simulink model "modelo_NL_DH_CL"  (R2025b)
settings: Solver=ode4  StartTime=0.0  StopTime=60  FixedStep=SampleTime  RelTol=1e-3
undefined symbols (not defined in the file): act, C_alt, C_phi, C_theta, C_vel, eng, h_ref, h_step_final, h_step_init, h_step_t, h_step_t2, h_step_t3, he, K_heading, Kp, Kq, Kr, psi_ref_final, psi_ref_init, psi_ref_t, psi_ref_t2, psi_ref_t3, tau_ref, theta_ref_clamp, TrimInput, Ue, Ve, VT_ref, VT_step_delta, VT_step_t, Xe
libraries: slpidlib x4
settings Model: Creator=anade  LastModifiedBy=kaue
settings SolverCC: ZeroCrossAlgorithm=Adaptive
settings DebuggingCC: AlgebraicLoopMsg=none  IgnoredZcDiagnostic=none

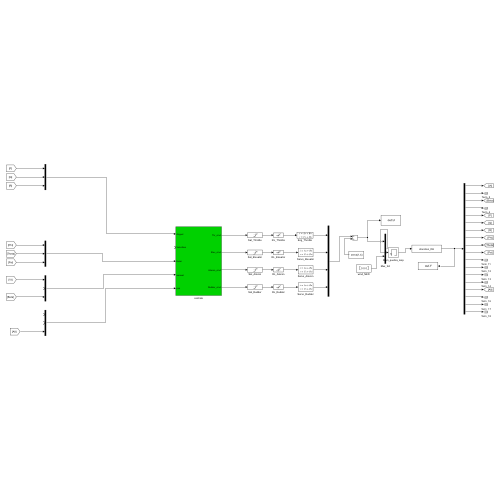
[thumbnail: Simulink's stored preview of the top-level diagram]
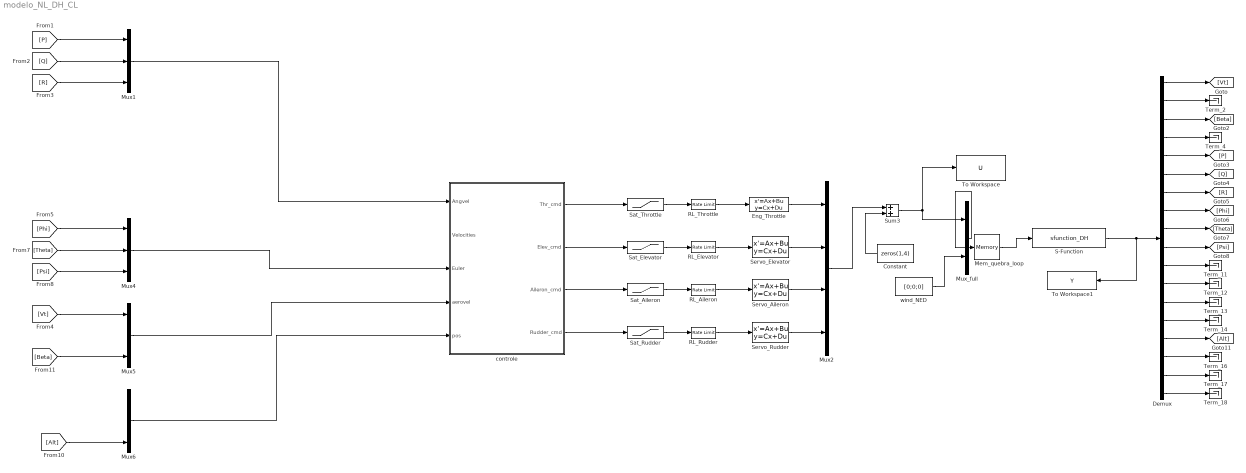
== system modelo_NL_DH_CL ==
  Constant : Constant  Value=zeros(1,4)
  Demux : Demux  Outputs=18
  Eng_Throttle : StateSpace  A=-1/eng.tau  B=1/eng.tau  D=0  InitialCondition=TrimInput(1)
  Mem_quebra_loop : Memory  Description=Quebra o loop algebrico da malha de controle atraves da S-function nivel-1 (que declara feedthrough direto em todas as entradas). Atraso de 1 passo (0.01 s) = comportamento do firmware real a 100 Hz, que atua com a medicao do ciclo anterior. IC = Ue (trim 7 entradas: 4 superficies + vento NED zero), sem transiente em t=0. Ganho medido: sim de 60 s caiu de ~100 s para ~9 s, diferenca de trajetoria <=0.18 deg / 1.1 cm na manobra agressiva (2026-06-09).  InitialCondition=Ue
  Mux{1,4..6} (4 alike) : Mux  Inputs=3
  Mux2 : Mux
  Mux_full : Mux  Inputs=2
  RL_Aileron : RateLimiter  RisingSlewLimit=act.rate  FallingSlewLimit=-act.rate  InitialCondition=TrimInput(3)
  RL_Elevator : RateLimiter  RisingSlewLimit=act.rate  FallingSlewLimit=-act.rate  InitialCondition=TrimInput(2)
  RL_Rudder : RateLimiter  RisingSlewLimit=act.rate  FallingSlewLimit=-act.rate  InitialCondition=TrimInput(4)
  RL_Throttle : RateLimiter  RisingSlewLimit=eng.rate  FallingSlewLimit=-eng.rate  InitialCondition=TrimInput(1)
  S-Function : S-Function  FunctionName=sfunction_DH  Parameters=Xe  SFunctionDeploymentMode=off  EnableBusSupport=off
  Sat_Aileron : Saturate  UpperLimit=0.4363  LowerLimit=-0.4363
  Sat_Elevator : Saturate  UpperLimit=0.4363  LowerLimit=-0.4363
  Sat_Rudder : Saturate  UpperLimit=0.4363  LowerLimit=-0.4363
  Sat_Throttle : Saturate  UpperLimit=1  LowerLimit=0
  Servo_Aileron : StateSpace  A=-act.bw  B=act.bw  D=0  InitialCondition=TrimInput(3)
  Servo_Elevator : StateSpace  A=-act.bw  B=act.bw  D=0  InitialCondition=TrimInput(2)
  Servo_Rudder : StateSpace  A=-act.bw  B=act.bw  D=0  InitialCondition=TrimInput(4)
  Sum3 : Sum
  Term_{2,4,11..14,16..18} (9 alike) : Terminator
  To Workspace : ToWorkspace  VariableName=U  SaveFormat=Structure With Time  SampleTime=-1
  To Workspace1 : ToWorkspace  VariableName=Y  SaveFormat=Structure With Time  SampleTime=-1
  controle : Subsystem
  wind_NED : Constant  Value=[0;0;0]
  wires:
  [Theta] -> Mux4/2
  Mux1/1 -> controle/1(Angvel)
  [Alt] -> Mux6/3
  [P] -> Mux1/1
  Mux4/1 -> controle/3(Euler)
  [R] -> Mux1/3
  [Phi] -> Mux4/1
  Mux6/1 -> controle/5(pos)
  [Q] -> Mux1/2
  Mux5/1 -> controle/4(aerovel)
  [Psi] -> Mux4/3
  [Beta] -> Mux5/3
  [Vt] -> Mux5/1
  controle/1(Thr_cmd) -> Sat_Throttle/1
  controle/2(Elev_cmd) -> Sat_Elevator/1
  controle/3(Aileron_cmd) -> Sat_Aileron/1
  controle/4(Rudder_cmd) -> Sat_Rudder/1
  Mux2/1 -> Sum3/1
  Constant/1 -> Sum3/2
  Sum3/1 -> Mux_full/1, To Workspace/1
  wind_NED/1 -> Mux_full/2
  S-Function/1 -> Demux/1, To Workspace1/1
  Demux/1 -> [Vt]
  Demux/2 -> Term_2/1
  Demux/3 -> [Beta]
  Demux/4 -> Term_4/1
  Demux/5 -> [P]
  Demux/6 -> [Q]
  Demux/7 -> [R]
  Demux/8 -> [Phi]
  Demux/9 -> [Theta]
  Demux/10 -> [Psi]
  Demux/11 -> Term_11/1
  Demux/12 -> Term_12/1
  Demux/13 -> Term_13/1
  Demux/14 -> Term_14/1
  Demux/15 -> [Alt]
  Demux/16 -> Term_16/1
  Demux/17 -> Term_17/1
  Demux/18 -> Term_18/1
  Mux_full/1 -> Mem_quebra_loop/1
  Mem_quebra_loop/1 -> S-Function/1
  Sat_Elevator/1 -> RL_Elevator/1
  Sat_Aileron/1 -> RL_Aileron/1
  Sat_Rudder/1 -> RL_Rudder/1
  RL_Elevator/1 -> Servo_Elevator/1
  Servo_Elevator/1 -> Mux2/2
  RL_Aileron/1 -> Servo_Aileron/1
  Servo_Aileron/1 -> Mux2/3
  RL_Rudder/1 -> Servo_Rudder/1
  Servo_Rudder/1 -> Mux2/4
  Sat_Throttle/1 -> RL_Throttle/1
  RL_Throttle/1 -> Eng_Throttle/1
  Eng_Throttle/1 -> Mux2/1

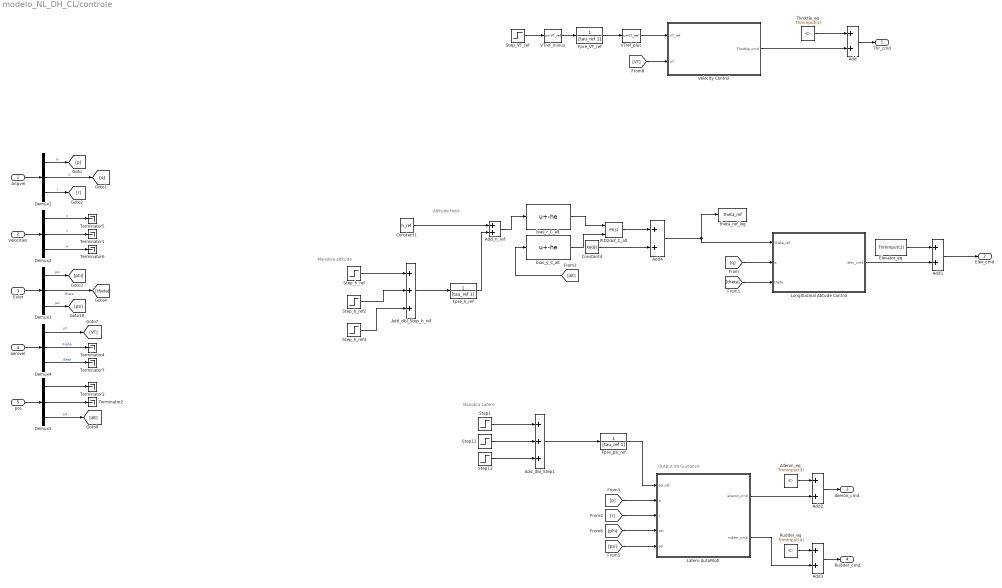
== system modelo_NL_DH_CL/controle ==
  note: Manobra
      | Latero
  note: Manobra
      | altitude
  note: Altitude Hold
  note: Output do Guidance
  Angvel : Inport
  Velocities : Inport  Port=2
  Euler : Inport  Port=3
  aerovel : Inport  Port=4
  pos : Inport  Port=5
  Add{,1..4} (5 alike) : Sum
  Add_dbl_Step1 : Sum  Inputs=+++
  Add_dbl_Step_h_ref : Sum  Inputs=+++
  Add_h_ref : Sum
  Aileron_eq : Constant  Value=TrimInput(3)
  Constant1 : Constant  Value=h_ref
  Constant4 : Constant  Value=Xe(8)
  Demux{1..5} (5 alike) : Demux  Outputs=3
  Elevator_eq : Constant  Value=TrimInput(2)
  Fpre_VT_ref : TransferFcn  Denominator=[tau_ref 1]
  Fpre_h_ref : TransferFcn  Denominator=[tau_ref 1]
  Fpre_psi_ref : TransferFcn  Denominator=[tau_ref 1]
  Latero AutoPilotl : Subsystem
  Longitudinal Atitude Control : Subsystem
  PID2dof_C_alt : slpidlib/PID Controller (2DOF)  Controller=PI  Form=Parallel  TimeDomain=Continuous-time  UseExternalTs=off  SampleTime=-1  IntegratorMethod=Forward Euler  FilterMethod=Forward Euler  ControllerParametersSource=internal  P=C_alt.Kp  I=C_alt.Ki  UseKiTs=off  D=0  UseExternalDerivativeSource=off  N=100  UseFilter=on  b=0  c=1  TunerSelectOption=Transfer Function Based (PID Tuner App)  InitialConditionSource=internal  InitialConditionForIntegrator=0  InitialConditionForFilter=0  DifferentiatorICPrevScaledInput=0  ExternalReset=none  TrackingMode=off  Kt=1  LimitOutput=on  SatLimitsSource=internal  UpperSaturationLimit=theta_ref_clamp(2)  LowerSaturationLimit=theta_ref_clamp(1)  LinearizeAsGain=on  AntiWindupMode=clamping  Kb=1  LimitIntegrator=off  UpperIntegratorSaturationLimit=inf  LowerIntegratorSaturationLimit=-inf  POutMin=[]  POutMax=[]  IOutMin=[]  IOutMax=[]  DOutMin=[]  DOutMax=[]  NOutMin=[]  NOutMax=[]  bOutMin=[]  bOutMax=[]  cOutMin=[]  cOutMax=[]  SumOutMin=[]  SumOutMax=[]  SaturationOutMin=[]  SaturationOutMax=[]  PParamMin=[]  PParamMax=[]  IParamMin=[]  IParamMax=[]  DParamMin=[]  DParamMax=[]  NParamMin=[]  NParamMax=[]  bParamMin=[]  bParamMax=[]  cParamMin=[]  cParamMax=[]  KbParamMin=[]  KbParamMax=[]  KtParamMin=[]  KtParamMax=[]  KbOutMin=[]  KbOutMax=[]  KtOutMin=[]  KtOutMax=[]  IntegratorOutMin=[]  IntegratorOutMax=[]  FilterOutMin=[]  FilterOutMax=[]  SumI1OutMin=[]  SumI1OutMax=[]  SumI2OutMin=[]  SumI2OutMax=[]  SumI3OutMin=[]  SumI3OutMax=[]  SumI4OutMin=[]  SumI4OutMax=[]  SumDOutMin=[]  SumDOutMax=[]  Sum1OutMin=[]  Sum1OutMax=[]  Sum2OutMin=[]  Sum2OutMax=[]  Sum3OutMin=[]  Sum3OutMax=[]  DifferentiatorOutMin=[]  DifferentiatorOutMax=[]  FilterDiffOutCoefMin=[]  FilterDiffOutCoefMax=[]  ReciprocalOutMin=[]  ReciprocalOutMax=[]  SumDenOutMin=[]  SumDenOutMax=[]  SumNumOutMin=[]  SumNumOutMax=[]  DivideOutMin=[]  DivideOutMax=[]  UdiffTsProdOutMin=[]  UdiffTsProdOutMax=[]  NTsProdOutMin=[]  NTsProdOutMax=[]  UintegralTsProdOutMin=[]  UintegralTsProdOutMax=[]  UngainTsProdOutMin=[]  UngainTsProdOutMax=[]  ClampingZeroOutDataTypeStr=Inherit: Inherit via back propagation  ClampingZeroOutMin=[]  ClampingZeroOutMax=[]  FilterDenConstantOutDataTypeStr=Inherit: Inherit via back propagation  FilterDenConstantOutMin=[]  FilterDenConstantOutMax=[]  PCopyOutDataTypeStr=Inherit: Inherit via back propagation  PCopyOutMin=[]  PCopyOutMax=[]  NCopyOutDataTypeStr=Inherit: Inherit via back propagation  NCopyOutMin=[]  NCopyOutMax=[]  IntegratorContinuousStateAttributes=''  IntegratorStateMustResolveToSignalObject=off  IntegratorRTWStateStorageClass=Auto  FilterContinuousStateAttributes=''  FilterStateMustResolveToSignalObject=off  FilterRTWStateStorageClass=Auto  ParallelPVariant=InternalParameters  IdealPVariant=Disabled  IVariant=InternalParameters  DVariant=Disabled  bVariant=InternalParameters  cVariant=Disabled  IntegratorVariant=Continuous  SatVariant=Enabled  AWVariant=ContClampingParallel  PCopyVariant=Disabled  TRVariant=Disabled  FdbkBlocksVariant=Forward  IdealPFdbkVariant=Disabled  SatFdbkVariant=Disabled  DerivativeFilterVariant=Disabled  NVariant=Disabled  NCopyVariant=Disabled_SignalSpec  FilterICVariant=Disabled  IntegratorICVariant=InternalICs  ExternalResetVariant=Disabled  TRSumVariant=Passthrough  SumFdbkVariant=Disabled  SumVariant=Sum_PI  TsampFilterVariant=InternalTs  TsampNgainVariant=Passthrough  TsampIntegralVariant=Disabled_SignalSpec  ExternalSaturationOutDataTypeStr=Inherit: Same as second input  DerivativeSourceVariant=Disabled  PreIntVariant=InternalPreInt
  Rudder_eq : Constant  Value=TrimInput(4)
  Step1 : Step  Time=psi_ref_t  Before=psi_ref_init  After=psi_ref_final  SampleTime=0
  Step12 : Step  Time=psi_ref_t2  After=-2*psi_ref_final  SampleTime=0
  Step13 : Step  Time=psi_ref_t3  After=psi_ref_final  SampleTime=0
  Step_VT_ref : Step  Time=VT_step_t  Before=VT_ref  After=VT_ref+VT_step_delta  SampleTime=0
  Step_h_ref : Step  Time=h_step_t  Before=h_step_init  After=h_step_final  SampleTime=0
  Step_h_ref2 : Step  Time=h_step_t2  After=-2*h_step_final  SampleTime=0
  Step_h_ref3 : Step  Time=h_step_t3  After=h_step_final  SampleTime=0
  Terminator{1..7} (7 alike) : Terminator
  Throttle_eq : Constant  Value=TrimInput(1)
  VTref_minus : Bias  Bias=-VT_ref
  VTref_plus : Bias  Bias=VT_ref
  Velocity Control : Subsystem
  bias_r_C_alt : Bias  Bias=-he  SaturateOnIntegerOverflow=off
  bias_y_C_alt : Bias  Bias=-he  SaturateOnIntegerOverflow=off
  theta_ref_log : ToWorkspace  VariableName=theta_ref  SaveFormat=Structure With Time  SampleTime=-1
  Thr_cmd : Outport
  Elev_cmd : Outport  Port=2
  Aileron_cmd : Outport  Port=3
  Rudder_cmd : Outport  Port=4
  wires:
  Angvel/1 -> Demux1/1
  Velocities/1 -> Demux2/1
  Demux1/1 -> [p]  "p"
  Demux1/2 -> [q]  "q"
  Demux1/3 -> [r]  "r"
  Euler/1 -> Demux3/1
  Demux3/3 -> [psi]  "psi"
  Demux3/1 -> [phi]  "phi"
  Demux3/2 -> [theta]  "theta"
  Demux2/3 -> Terminator6/1  "w"
  Demux2/1 -> Terminator5/1  "u"
  Demux2/2 -> Terminator1/1  "v"
  [theta] -> Longitudinal Atitude Control/3(theta)
  aerovel/1 -> Demux4/1
  Demux4/1 -> [VT]  "VT"
  Demux4/2 -> Terminator4/1  "Alpha"
  Demux4/3 -> Terminator7/1  "Beta"
  [q] -> Longitudinal Atitude Control/2(q)
  [VT] -> Velocity Control/2(VT)
  pos/1 -> Demux5/1
  Demux5/3 -> [alt]  "alt"
  Demux5/2 -> Terminator2/1
  Demux5/1 -> Terminator3/1
  [p] -> Latero AutoPilotl/2(p)
  [r] -> Latero AutoPilotl/3(r)
  [psi] -> Latero AutoPilotl/5(psi)
  [phi] -> Latero AutoPilotl/4(phi)
  Constant4/1 -> Add4/2
  Add1/1 -> Elev_cmd/1
  Longitudinal Atitude Control/1(elev_cmd) -> Add1/2
  Add/1 -> Thr_cmd/1
  Velocity Control/1(Throttle_cmd) -> Add/2
  Latero AutoPilotl/1(aileron_cmd) -> Add2/2
  Elevator_eq/1 -> Add1/1
  Rudder_eq/1 -> Add3/1
  Aileron_eq/1 -> Add2/1
  Latero AutoPilotl/2(rudder_cmd) -> Add3/2
  Add2/1 -> Aileron_cmd/1
  Add3/1 -> Rudder_cmd/1
  Throttle_eq/1 -> Add/1
  Step_VT_ref/1 -> VTref_minus/1
  Add4/1 -> theta_ref_log/1, Longitudinal Atitude Control/1(Theta_ref)
  Constant1/1 -> Add_h_ref/1
  Step_h_ref/1 -> Add_dbl_Step_h_ref/1
  Step_h_ref2/1 -> Add_dbl_Step_h_ref/2
  Step_h_ref3/1 -> Add_dbl_Step_h_ref/3
  Step1/1 -> Add_dbl_Step1/1
  Step12/1 -> Add_dbl_Step1/2
  Step13/1 -> Add_dbl_Step1/3
  Add_dbl_Step_h_ref/1 -> Fpre_h_ref/1
  Fpre_h_ref/1 -> Add_h_ref/2
  Add_dbl_Step1/1 -> Fpre_psi_ref/1
  Fpre_psi_ref/1 -> Latero AutoPilotl/1(psi_ref)
  VTref_minus/1 -> Fpre_VT_ref/1
  Fpre_VT_ref/1 -> VTref_plus/1
  VTref_plus/1 -> Velocity Control/1(VT_ref)
  Add_h_ref/1 -> bias_r_C_alt/1
  [alt] -> bias_y_C_alt/1
  bias_r_C_alt/1 -> PID2dof_C_alt/1
  bias_y_C_alt/1 -> PID2dof_C_alt/2
  PID2dof_C_alt/1 -> Add4/1

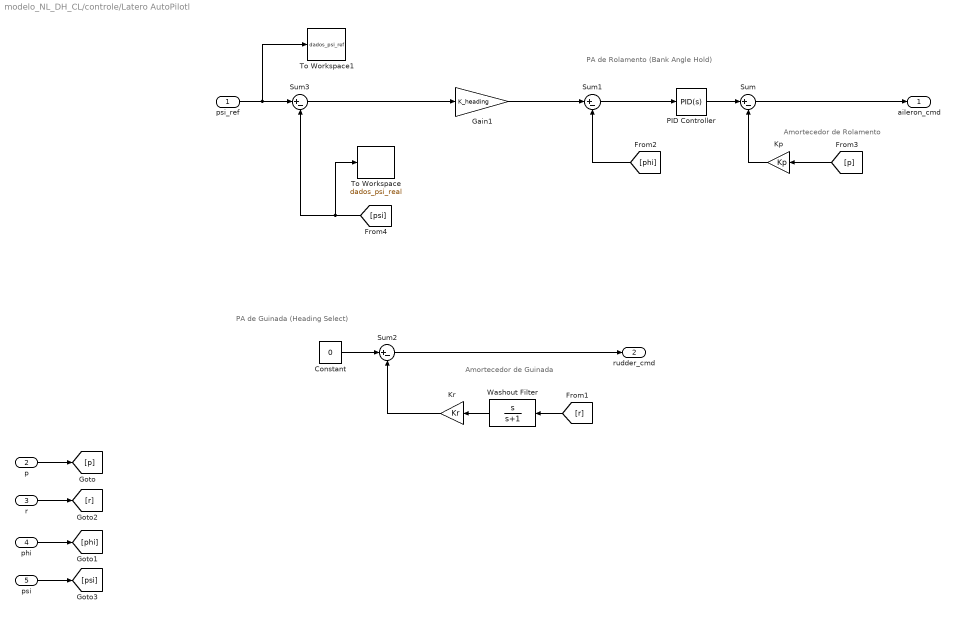
== system modelo_NL_DH_CL/controle/Latero AutoPilotl ==
  note: PA de Rolamento (Bank Angle Hold)
  note: Amortecedor de Rolamento
  note: Amortecedor de Guinada
  note: PA de Guinada (Heading Select)
  psi_ref : Inport
  p : Inport  Port=2
  r : Inport  Port=3
  phi : Inport  Port=4
  psi : Inport  Port=5
  Constant : Constant  Value=0
  Gain1 : Gain  Gain=K_heading
  Kp : Gain  Gain=Kp
  Kr : Gain  Gain=Kr
  PID Controller : slpidlib/PID Controller  Controller=PID  Form=Parallel  TimeDomain=Continuous-time  UseExternalTs=off  SampleTime=-1  IntegratorMethod=Forward Euler  FilterMethod=Forward Euler  ControllerParametersSource=internal  P=C_phi.Kp  I=C_phi.Ki  UseKiTs=off  D=C_phi.Kd  UseExternalDerivativeSource=off  N=C_phi.N  UseFilter=on  TunerSelectOption=Transfer Function Based (PID Tuner App)  InitialConditionSource=internal  InitialConditionForIntegrator=0  InitialConditionForFilter=0  DifferentiatorICPrevScaledInput=0  ExternalReset=none  TrackingMode=off  Kt=1  LimitOutput=on  SatLimitsSource=internal  UpperSaturationLimit=0.4363  LowerSaturationLimit=-0.4363  LinearizeAsGain=on  AntiWindupMode=clamping  Kb=1  LimitIntegrator=off  UpperIntegratorSaturationLimit=inf  LowerIntegratorSaturationLimit=-inf  POutMin=[]  POutMax=[]  IOutMin=[]  IOutMax=[]  DOutMin=[]  DOutMax=[]  NOutMin=[]  NOutMax=[]  SumOutMin=[]  SumOutMax=[]  SaturationOutMin=[]  SaturationOutMax=[]  PParamMin=[]  PParamMax=[]  IParamMin=[]  IParamMax=[]  DParamMin=[]  DParamMax=[]  NParamMin=[]  NParamMax=[]  KbParamMin=[]  KbParamMax=[]  KtParamMin=[]  KtParamMax=[]  KbOutMin=[]  KbOutMax=[]  KtOutMin=[]  KtOutMax=[]  IntegratorOutMin=[]  IntegratorOutMax=[]  FilterOutMin=[]  FilterOutMax=[]  SumI1OutMin=[]  SumI1OutMax=[]  SumI2OutMin=[]  SumI2OutMax=[]  SumI3OutMin=[]  SumI3OutMax=[]  SumI4OutMin=[]  SumI4OutMax=[]  SumDOutMin=[]  SumDOutMax=[]  DifferentiatorOutMin=[]  DifferentiatorOutMax=[]  FilterDiffOutCoefMin=[]  FilterDiffOutCoefMax=[]  ReciprocalOutMin=[]  ReciprocalOutMax=[]  SumDenOutMin=[]  SumDenOutMax=[]  SumNumOutMin=[]  SumNumOutMax=[]  DivideOutMin=[]  DivideOutMax=[]  UdiffTsProdOutMin=[]  UdiffTsProdOutMax=[]  NTsProdOutMin=[]  NTsProdOutMax=[]  UintegralTsProdOutMin=[]  UintegralTsProdOutMax=[]  UngainTsProdOutMin=[]  UngainTsProdOutMax=[]  ClampingZeroOutDataTypeStr=Inherit: Inherit via back propagation  ClampingZeroOutMin=[]  ClampingZeroOutMax=[]  FilterDenConstantOutDataTypeStr=Inherit: Inherit via back propagation  FilterDenConstantOutMin=[]  FilterDenConstantOutMax=[]  PCopyOutDataTypeStr=Inherit: Inherit via back propagation  PCopyOutMin=[]  PCopyOutMax=[]  NCopyOutDataTypeStr=Inherit: Inherit via back propagation  NCopyOutMin=[]  NCopyOutMax=[]  IntegratorContinuousStateAttributes=''  IntegratorStateMustResolveToSignalObject=off  IntegratorRTWStateStorageClass=Auto  FilterContinuousStateAttributes=''  FilterStateMustResolveToSignalObject=off  FilterRTWStateStorageClass=Auto  ParallelPVariant=InternalParameters  IdealPVariant=Disabled  IVariant=InternalParameters  DVariant=InternalParameters  IntegratorVariant=Continuous  SatVariant=Enabled  AWVariant=ContClampingParallel  PCopyVariant=Disabled  TRVariant=Disabled  FdbkBlocksVariant=Forward  IdealPFdbkVariant=Disabled  SatFdbkVariant=Disabled  DerivativeFilterVariant=ContFilter  NVariant=InternalParameters  NCopyVariant=Disabled  FilterICVariant=InternalICsFilter  IntegratorICVariant=InternalICs  ExternalResetVariant=Disabled  TRSumVariant=Passthrough  SumFdbkVariant=Disabled  SumVariant=Sum_PID  TsampFilterVariant=InternalTs  TsampNgainVariant=Passthrough  TsampIntegralVariant=Disabled_SignalSpec  ExternalSaturationOutDataTypeStr=Inherit: Same as second input  DerivativeSourceVariant=ErrorSignal  PreIntVariant=InternalPreInt
  Sum{,1..3} (4 alike) : Sum  Inputs=|+-
  To Workspace : ToWorkspace  VariableName=dados_psi_real  SaveFormat=Timeseries  SampleTime=-1
      settings: Save2DSignal=2-D array (concatenate along first dimension)
  To Workspace1 : ToWorkspace  VariableName=dados_psi_ref  SaveFormat=Timeseries  SampleTime=-1
      settings: Save2DSignal=2-D array (concatenate along first dimension)
  Washout Filter : TransferFcn  Numerator=[1 0]  Denominator=[1 1]
  aileron_cmd : Outport
  rudder_cmd : Outport  Port=2
  wires:
  [p] -> Kp/1
  [phi] -> Sum1/2
  Kp/1 -> Sum/2
  PID Controller/1 -> Sum/1
  p/1 -> [p]
  [r] -> Washout Filter/1
  Kr/1 -> Sum2/2
  r/1 -> [r]
  Washout Filter/1 -> Kr/1
  phi/1 -> [phi]
  psi/1 -> [psi]
  Sum3/1 -> Gain1/1
  [psi] -> Sum3/2, To Workspace/1
  psi_ref/1 -> Sum3/1, To Workspace1/1
  Sum2/1 -> rudder_cmd/1
  Constant/1 -> Sum2/1
  Gain1/1 -> Sum1/1
  Sum/1 -> aileron_cmd/1
  Sum1/1 -> PID Controller/1

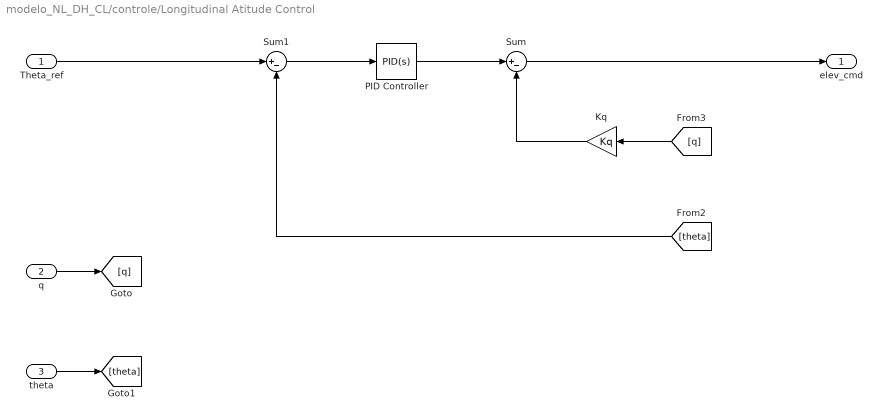
== system modelo_NL_DH_CL/controle/Longitudinal Atitude Control ==
  Theta_ref : Inport
  q : Inport  Port=2
  theta : Inport  Port=3
  Kq : Gain  Gain=Kq
  PID Controller : slpidlib/PID Controller  Controller=PID  Form=Parallel  TimeDomain=Continuous-time  UseExternalTs=off  SampleTime=-1  IntegratorMethod=Forward Euler  FilterMethod=Forward Euler  ControllerParametersSource=internal  P=C_theta.Kp  I=C_theta.Ki  UseKiTs=off  D=C_theta.Kd  UseExternalDerivativeSource=off  N=C_theta.N  UseFilter=on  TunerSelectOption=Transfer Function Based (PID Tuner App)  InitialConditionSource=internal  InitialConditionForIntegrator=0  InitialConditionForFilter=0  DifferentiatorICPrevScaledInput=0  ExternalReset=none  TrackingMode=off  Kt=1  LimitOutput=on  SatLimitsSource=internal  UpperSaturationLimit=0.4363  LowerSaturationLimit=-0.4363  LinearizeAsGain=on  AntiWindupMode=clamping  Kb=1  LimitIntegrator=off  UpperIntegratorSaturationLimit=inf  LowerIntegratorSaturationLimit=-inf  POutMin=[]  POutMax=[]  IOutMin=[]  IOutMax=[]  DOutMin=[]  DOutMax=[]  NOutMin=[]  NOutMax=[]  SumOutMin=[]  SumOutMax=[]  SaturationOutMin=[]  SaturationOutMax=[]  PParamMin=[]  PParamMax=[]  IParamMin=[]  IParamMax=[]  DParamMin=[]  DParamMax=[]  NParamMin=[]  NParamMax=[]  KbParamMin=[]  KbParamMax=[]  KtParamMin=[]  KtParamMax=[]  KbOutMin=[]  KbOutMax=[]  KtOutMin=[]  KtOutMax=[]  IntegratorOutMin=[]  IntegratorOutMax=[]  FilterOutMin=[]  FilterOutMax=[]  SumI1OutMin=[]  SumI1OutMax=[]  SumI2OutMin=[]  SumI2OutMax=[]  SumI3OutMin=[]  SumI3OutMax=[]  SumI4OutMin=[]  SumI4OutMax=[]  SumDOutMin=[]  SumDOutMax=[]  DifferentiatorOutMin=[]  DifferentiatorOutMax=[]  FilterDiffOutCoefMin=[]  FilterDiffOutCoefMax=[]  ReciprocalOutMin=[]  ReciprocalOutMax=[]  SumDenOutMin=[]  SumDenOutMax=[]  SumNumOutMin=[]  SumNumOutMax=[]  DivideOutMin=[]  DivideOutMax=[]  UdiffTsProdOutMin=[]  UdiffTsProdOutMax=[]  NTsProdOutMin=[]  NTsProdOutMax=[]  UintegralTsProdOutMin=[]  UintegralTsProdOutMax=[]  UngainTsProdOutMin=[]  UngainTsProdOutMax=[]  ClampingZeroOutDataTypeStr=Inherit: Inherit via back propagation  ClampingZeroOutMin=[]  ClampingZeroOutMax=[]  FilterDenConstantOutDataTypeStr=Inherit: Inherit via back propagation  FilterDenConstantOutMin=[]  FilterDenConstantOutMax=[]  PCopyOutDataTypeStr=Inherit: Inherit via back propagation  PCopyOutMin=[]  PCopyOutMax=[]  NCopyOutDataTypeStr=Inherit: Inherit via back propagation  NCopyOutMin=[]  NCopyOutMax=[]  IntegratorContinuousStateAttributes=''  IntegratorStateMustResolveToSignalObject=off  IntegratorRTWStateStorageClass=Auto  FilterContinuousStateAttributes=''  FilterStateMustResolveToSignalObject=off  FilterRTWStateStorageClass=Auto  ParallelPVariant=InternalParameters  IdealPVariant=Disabled  IVariant=InternalParameters  DVariant=InternalParameters  IntegratorVariant=Continuous  SatVariant=Enabled  AWVariant=ContClampingParallel  PCopyVariant=Disabled  TRVariant=Disabled  FdbkBlocksVariant=Forward  IdealPFdbkVariant=Disabled  SatFdbkVariant=Disabled  DerivativeFilterVariant=ContFilter  NVariant=InternalParameters  NCopyVariant=Disabled  FilterICVariant=InternalICsFilter  IntegratorICVariant=InternalICs  ExternalResetVariant=Disabled  TRSumVariant=Passthrough  SumFdbkVariant=Disabled  SumVariant=Sum_PID  TsampFilterVariant=InternalTs  TsampNgainVariant=Passthrough  TsampIntegralVariant=Disabled_SignalSpec  ExternalSaturationOutDataTypeStr=Inherit: Same as second input  DerivativeSourceVariant=ErrorSignal  PreIntVariant=InternalPreInt
  Sum : Sum  Inputs=|+-
  Sum1 : Sum  Inputs=|+-
  elev_cmd : Outport
  wires:
  Sum1/1 -> PID Controller/1
  Sum/1 -> elev_cmd/1
  [q] -> Kq/1
  [theta] -> Sum1/2
  Kq/1 -> Sum/2
  PID Controller/1 -> Sum/1
  theta/1 -> [theta]
  q/1 -> [q]
  Theta_ref/1 -> Sum1/1

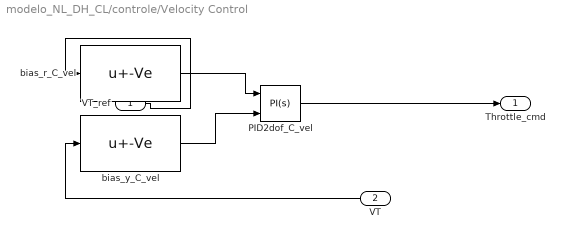
== system modelo_NL_DH_CL/controle/Velocity Control ==
  VT_ref : Inport
  VT : Inport  Port=2
  PID2dof_C_vel : slpidlib/PID Controller (2DOF)  Controller=PI  Form=Parallel  TimeDomain=Continuous-time  UseExternalTs=off  SampleTime=-1  IntegratorMethod=Forward Euler  FilterMethod=Forward Euler  ControllerParametersSource=internal  P=C_vel.Kp  I=C_vel.Ki  UseKiTs=off  D=0  UseExternalDerivativeSource=off  N=100  UseFilter=on  b=0  c=1  TunerSelectOption=Transfer Function Based (PID Tuner App)  InitialConditionSource=internal  InitialConditionForIntegrator=0  InitialConditionForFilter=0  DifferentiatorICPrevScaledInput=0  ExternalReset=none  TrackingMode=off  Kt=1  LimitOutput=on  SatLimitsSource=internal  UpperSaturationLimit=0.51  LowerSaturationLimit=-0.49  LinearizeAsGain=on  AntiWindupMode=clamping  Kb=1  LimitIntegrator=off  UpperIntegratorSaturationLimit=inf  LowerIntegratorSaturationLimit=-inf  POutMin=[]  POutMax=[]  IOutMin=[]  IOutMax=[]  DOutMin=[]  DOutMax=[]  NOutMin=[]  NOutMax=[]  bOutMin=[]  bOutMax=[]  cOutMin=[]  cOutMax=[]  SumOutMin=[]  SumOutMax=[]  SaturationOutMin=[]  SaturationOutMax=[]  PParamMin=[]  PParamMax=[]  IParamMin=[]  IParamMax=[]  DParamMin=[]  DParamMax=[]  NParamMin=[]  NParamMax=[]  bParamMin=[]  bParamMax=[]  cParamMin=[]  cParamMax=[]  KbParamMin=[]  KbParamMax=[]  KtParamMin=[]  KtParamMax=[]  KbOutMin=[]  KbOutMax=[]  KtOutMin=[]  KtOutMax=[]  IntegratorOutMin=[]  IntegratorOutMax=[]  FilterOutMin=[]  FilterOutMax=[]  SumI1OutMin=[]  SumI1OutMax=[]  SumI2OutMin=[]  SumI2OutMax=[]  SumI3OutMin=[]  SumI3OutMax=[]  SumI4OutMin=[]  SumI4OutMax=[]  SumDOutMin=[]  SumDOutMax=[]  Sum1OutMin=[]  Sum1OutMax=[]  Sum2OutMin=[]  Sum2OutMax=[]  Sum3OutMin=[]  Sum3OutMax=[]  DifferentiatorOutMin=[]  DifferentiatorOutMax=[]  FilterDiffOutCoefMin=[]  FilterDiffOutCoefMax=[]  ReciprocalOutMin=[]  ReciprocalOutMax=[]  SumDenOutMin=[]  SumDenOutMax=[]  SumNumOutMin=[]  SumNumOutMax=[]  DivideOutMin=[]  DivideOutMax=[]  UdiffTsProdOutMin=[]  UdiffTsProdOutMax=[]  NTsProdOutMin=[]  NTsProdOutMax=[]  UintegralTsProdOutMin=[]  UintegralTsProdOutMax=[]  UngainTsProdOutMin=[]  UngainTsProdOutMax=[]  ClampingZeroOutDataTypeStr=Inherit: Inherit via back propagation  ClampingZeroOutMin=[]  ClampingZeroOutMax=[]  FilterDenConstantOutDataTypeStr=Inherit: Inherit via back propagation  FilterDenConstantOutMin=[]  FilterDenConstantOutMax=[]  PCopyOutDataTypeStr=Inherit: Inherit via back propagation  PCopyOutMin=[]  PCopyOutMax=[]  NCopyOutDataTypeStr=Inherit: Inherit via back propagation  NCopyOutMin=[]  NCopyOutMax=[]  IntegratorContinuousStateAttributes=''  IntegratorStateMustResolveToSignalObject=off  IntegratorRTWStateStorageClass=Auto  FilterContinuousStateAttributes=''  FilterStateMustResolveToSignalObject=off  FilterRTWStateStorageClass=Auto  ParallelPVariant=InternalParameters  IdealPVariant=Disabled  IVariant=InternalParameters  DVariant=Disabled  bVariant=InternalParameters  cVariant=Disabled  IntegratorVariant=Continuous  SatVariant=Enabled  AWVariant=ContClampingParallel  PCopyVariant=Disabled  TRVariant=Disabled  FdbkBlocksVariant=Forward  IdealPFdbkVariant=Disabled  SatFdbkVariant=Disabled  DerivativeFilterVariant=Disabled  NVariant=Disabled  NCopyVariant=Disabled_SignalSpec  FilterICVariant=Disabled  IntegratorICVariant=InternalICs  ExternalResetVariant=Disabled  TRSumVariant=Passthrough  SumFdbkVariant=Disabled  SumVariant=Sum_PI  TsampFilterVariant=InternalTs  TsampNgainVariant=Passthrough  TsampIntegralVariant=Disabled_SignalSpec  ExternalSaturationOutDataTypeStr=Inherit: Same as second input  DerivativeSourceVariant=Disabled  PreIntVariant=InternalPreInt
  bias_r_C_vel : Bias  Bias=-Ve  SaturateOnIntegerOverflow=off
  bias_y_C_vel : Bias  Bias=-Ve  SaturateOnIntegerOverflow=off
  Throttle_cmd : Outport
  wires:
  VT_ref/1 -> bias_r_C_vel/1
  VT/1 -> bias_y_C_vel/1
  bias_r_C_vel/1 -> PID2dof_C_vel/1
  bias_y_C_vel/1 -> PID2dof_C_vel/2
  PID2dof_C_vel/1 -> Throttle_cmd/1
